simulink model "strong_wind"  (R2019b)
settings: Solver=VariableStepAuto  StartTime=0.0  StopTime=140  RelTol=1e-3
undefined symbols (not defined in the file): drywind, GreensiteLPV
libraries: simulink x2, cstblocks x1
settings Model: Creator=Alessandro  LastModifiedBy=Alessandro

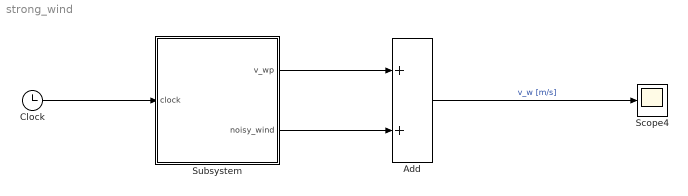
== system strong_wind ==
  Add : Sum
  Clock : Clock
  Scope4 : Scope
  Subsystem : Subsystem
  wires:
  Clock/1 -> Subsystem/1(clock)
  Add/1 -> Scope4/1  "v_w [m/s]"
  Subsystem/2(noisy_wind) -> Add/2
  Subsystem/1(v_wp) -> Add/1

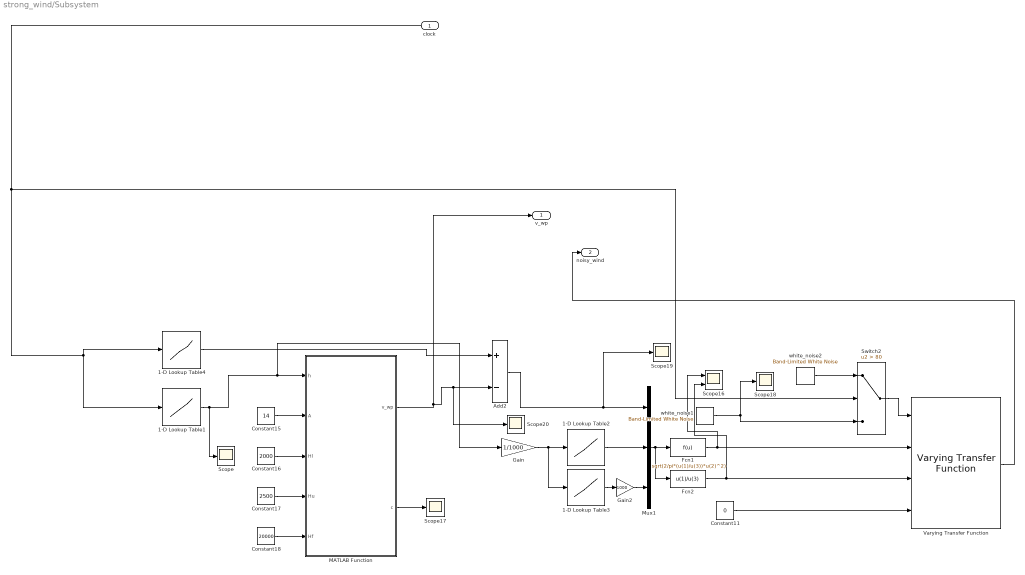
== system strong_wind/Subsystem ==
  clock : Inport
  1-D Lookup Table1 : Lookup_n-D  NumberOfTableDimensions=1  BreakpointsForDimension1=GreensiteLPV.h.Time  Table=GreensiteLPV.h.Data  InternalRulePriority=Speed  RndMeth=Simplest  InputSameDT=on
  1-D Lookup Table2 : Lookup_n-D  NumberOfTableDimensions=1  BreakpointsForDimension1=drywind.alt  Table=drywind.sigma.severe  InternalRulePriority=Speed  RndMeth=Simplest  InputSameDT=on
  1-D Lookup Table3 : Lookup_n-D  NumberOfTableDimensions=1  BreakpointsForDimension1=drywind.alt  Table=drywind.Lh  InternalRulePriority=Speed  RndMeth=Simplest  InputSameDT=on
  1-D Lookup Table4 : Lookup_n-D  NumberOfTableDimensions=1  BreakpointsForDimension1=GreensiteLPV.V.Time  Table=GreensiteLPV.V.Data  InternalRulePriority=Speed  RndMeth=Simplest  InputSameDT=on
  Add2 : Sum  Inputs=+-
  Constant11 : Constant  Value=0
  Constant15 : Constant  Value=14
  Constant16 : Constant  Value=2000
  Constant17 : Constant  Value=2500
  Constant18 : Constant  Value=20000
  Fcn1 : Fcn  Expr=sqrt(2/pi*(u(1)/u(3))*u(2)^2)
  Fcn2 : Fcn  Expr=u(1)/u(3)
  Gain : Gain  Gain=1/1000
  Gain2 : Gain  Gain=1000
  MATLAB Function : MATLAB Function  TreatAsAtomicUnit=on
  Mux1 : Mux  Inputs=3
  Scope{,17..20} (5 alike) : Scope
  Scope16 : Scope  NumInputPorts=2
  Switch2 : Switch  Criteria=u2 > Threshold  Threshold=80
  Varying Transfer Function : cstblocks/Linear Parameter Varying/Varying Transfer Function  N=1
      settings: SourceProductName=Control System Toolbox
  white_noise1 : simulink/Sources/Band-Limited White Noise  Cov=[1]  Ts=0.1  seed=22222
  white_noise2 : simulink/Sources/Band-Limited White Noise  Cov=[0.01]  Ts=0.1  seed=22222
  v_wp : Outport
  noisy_wind : Outport  Port=2
  wires:
  Add2/1 -> Mux1/1, Scope19/1
  1-D Lookup Table4/1 -> Add2/1
  MATLAB Function/1(v_wp) -> v_wp/1, Add2/2, Scope20/1
  Gain2/1 -> Mux1/3
  Mux1/1 -> Fcn1/1, Fcn2/1
  1-D Lookup Table1/1 -> Scope/1, MATLAB Function/1(h), Gain/1
  clock/1 -> 1-D Lookup Table1/1, 1-D Lookup Table4/1, Switch2/2
  Constant15/1 -> MATLAB Function/2(A)
  white_noise1/1 -> Switch2/3, Scope18/1
  Constant16/1 -> MATLAB Function/3(Hl)
  MATLAB Function/2(c) -> Scope17/1
  white_noise2/1 -> Switch2/1
  Switch2/1 -> Varying Transfer Function/1
  Fcn2/1 -> Varying Transfer Function/3, Scope16/2
  Constant11/1 -> Varying Transfer Function/4
  Varying Transfer Function/1 -> noisy_wind/1
  1-D Lookup Table3/1 -> Gain2/1
  Gain/1 -> 1-D Lookup Table2/1, 1-D Lookup Table3/1
  1-D Lookup Table2/1 -> Mux1/2
  Constant18/1 -> MATLAB Function/5(Hf)
  Constant17/1 -> MATLAB Function/4(Hu)
  Fcn1/1 -> Varying Transfer Function/2, Scope16/1

== matlab function strong_wind/Subsystem/MATLAB Function ==
  data: h input; v_wp output; A input; Hl input; Hu input; Hf input; c output
function [v_wp,c] = fcn(h,A,Hl,Hu,Hf)
    if h < Hl
        v_wp = 10*A*(((h/2000)^(0.9))-0.9*(h/Hl));
        c = 1;
    elseif h >= Hl & h <= Hf-Hu
        v_wp = A;
        c = 2;
    elseif h > Hf-Hu & h <=Hf
        v_wp = A/2*(1 - cos((pi/Hu)*(h-Hf)));
        c = 3;
    else 
        v_wp = 0;
        c = 4;
    end
